simulink model "OpenLoop"  (R2022b)
settings: Solver=ode1  StartTime=0.0  StopTime=10  FixedStep=0.002  RelTol=1e-3  EnableMultiTasking=on
values from neighbouring files (symbols this model uses):
  a = -1/tau    (= -50)    [data_modele.m]
  Ao = [a 0;1 0]    [data_modele.m]
  Aobis = [a 0 b;1 0 0;0 0 0]    [data_modele.m]
  b = context.isCodeGenTarget('rtw')    [DCMotor1Set.m]    (also in DCMotor2Set.m; Enc1Period.m; Enc1Read.m; data_modele.m = 2500)
  Bo = [b;0]    [data_modele.m]
  Bobis = [b;0;0]    [data_modele.m]
  Co = [0 1]    [data_modele.m]
  Cobis = [0 1 0]    [data_modele.m]
  k1 = K(1, 2)    [data_modele.m]
  k2 = K(1, 1)    [data_modele.m]
  Kb = 50    [data_modele.m]
  L = transpose(Lt)    [data_modele.m]
  Lbis = transpose(Lbist)    [data_modele.m]
undefined symbols (not defined in the file or in its folder): sigbuilder_block
libraries: simulink x2
settings Model: SimulationMode=external  ExtModeTrigDuration=2  VariantFading=off  Creator=Alex  LastModifiedBy=mtroislo
settings SolverCC: AlgebraicLoopSolver=TrustRegion
settings DataIOCC: SaveFormat=StructureWithTime  ReturnWorkspaceOutputs=off
settings OptimizationCC: PassReuseOutputArgsAs=Individual arguments  MaxStackSize=64  EfficientTunableParamExpr=on
settings DebuggingCC: ParameterTunabilityLossMsg=error  UnconnectedInputMsg=warning  UnconnectedOutputMsg=warning  UnconnectedLineMsg=warning  SFMachineParentedDataDiag=warning  ArithmeticOperatorsInVariantConditions=warning
settings HardwareCC: ProdBitPerInt=16  ProdBitPerPointer=16  ProdBitPerSizeT=16  ProdBitPerPtrDiffT=16  ProdLargestAtomicFloat=None  ProdWordSize=8  ProdHWDeviceType=Atmel->AVR
settings ModelReferenceCC: EnableRefExpFcnMdlSchedulingChecks=on
settings SFSimCC: SimUseLocalCustomCode=off  MATLABDynamicMemAlloc=off  CustomCodeUndefinedFunction=UseInterfaceOnly
settings RTWCC: Description=Embedded Coder  SystemTargetFile=ert.tlc  HardwareBoard=Arduino Mega 2560  TLCOptions=-aInlineSetEventsForThisBaseRateFcn=TLC_FALSE -aSuppressMultiTaskScheduler=TLC_FALSE -aRateBasedStepFcn=1  TemplateMakefile=ert_default_tmf  RTWUseLocalCustomCode=off  Toolchain=Arduino AVR  BuildConfiguration=Faster Runs  IncludeHyperlinkInReport=on  DLArmComputeVersion=19.05
settings CodeAppCC: ForceParamTrailComments=on  IgnoreCustomStorageClasses=off  OperatorAnnotations=on  SimulinkDataObjDesc=on  SFDataObjDesc=on  InsertBlockDesc=on
settings ERTTargetCC: SupportContinuousTime=on  SupportVariableSizeSignals=on

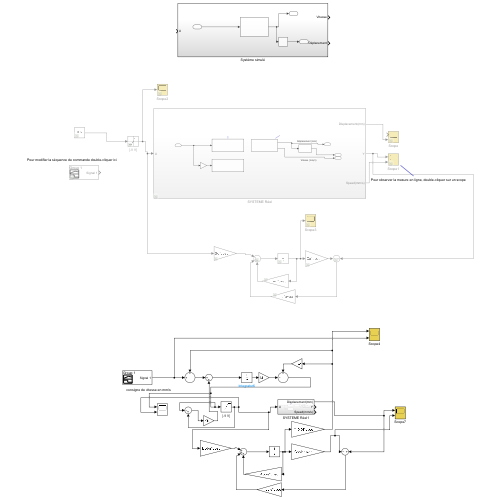
[thumbnail: Simulink's stored preview of the top-level diagram]
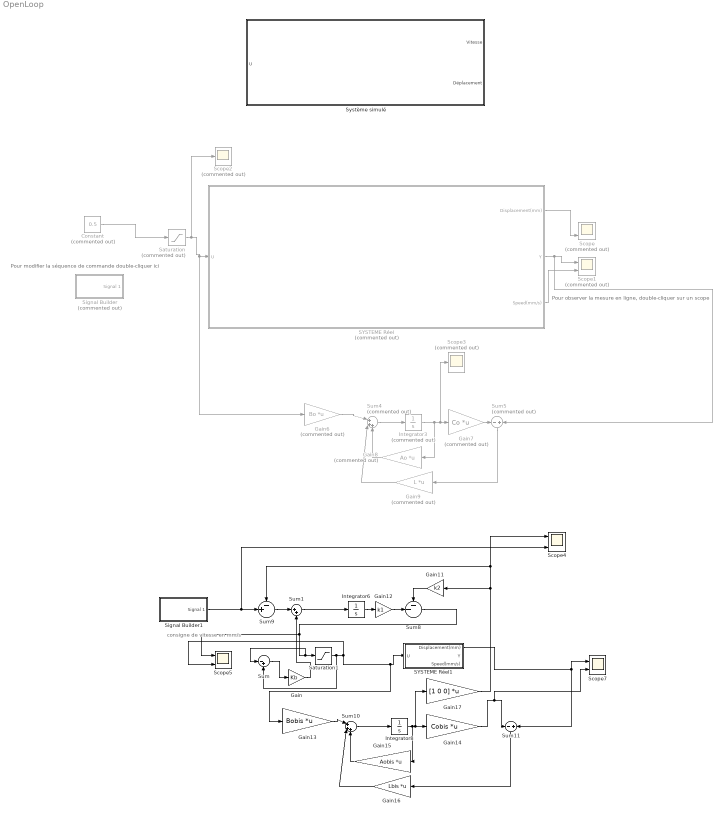
== system OpenLoop ==
  note: Pour observer la mesure en ligne, double-cliquer sur un scope
  note: Pour modifier la séquence de commande double-cliquer ici
  note: consigne de vitesse en mm/s
  Constant : Constant  Commented=on  Value=0.5
  Gain : Gain  Gain=Kb
  Gain11 : Gain  Gain=k2
  Gain12 : Gain  Gain=k1
  Gain13 : Gain  Gain=Bobis  Multiplication=Matrix(K*u) (u vector)
  Gain14 : Gain  Gain=Cobis  Multiplication=Matrix(K*u) (u vector)
  Gain15 : Gain  Gain=Aobis  Multiplication=Matrix(K*u) (u vector)
  Gain16 : Gain  Gain=Lbis  Multiplication=Matrix(K*u) (u vector)
  Gain17 : Gain  Gain=[1 0 0]  Multiplication=Matrix(K*u) (u vector)
  Gain6 : Gain  Commented=on  Gain=Bo  Multiplication=Matrix(K*u) (u vector)
  Gain7 : Gain  Commented=on  Gain=Co  Multiplication=Matrix(K*u) (u vector)
  Gain8 : Gain  Commented=on  Gain=Ao  Multiplication=Matrix(K*u) (u vector)
  Gain9 : Gain  Commented=on  Gain=L  Multiplication=Matrix(K*u) (u vector)
  Integrator3 : Integrator  Commented=on
  Integrator6 : Integrator
  Integrator8 : Integrator
  SYSTEME Réel : Subsystem  Commented=on
  SYSTEME Réel1 : Subsystem
  Saturation : Saturate  Commented=on  UpperLimit=9  LowerLimit=-9
      settings: AttributesFormatString=[%<LowerLimit> %<UpperLimit>]
  Saturation1 : Saturate  UpperLimit=9  LowerLimit=-9
      settings: AttributesFormatString=[%<LowerLimit> %<UpperLimit>]
  Scope : Scope  Commented=on  NumInputPorts=2
  Scope1 : Scope  Commented=on  NumInputPorts=2
  Scope2 : Scope  Commented=on
  Scope3 : Scope  Commented=on
  Scope4 : Scope  NumInputPorts=2
  Scope5 : Scope  NumInputPorts=2
  Scope7 : Scope  NumInputPorts=2
  Signal Builder : Subsystem  Tag=STV Subsys  Commented=on  LoadFcn=sigbuilder_block('load');  StartFcn=sigbuilder_block('start');  StopFcn=sigbuilder_block('stop');  ClipboardFcn=sigbuilder_block('clipboard');  mask(Sigbuilder block){tuvar=[0:10]}
      mask help: Simulink:masks:SigbuilderBlock_MD
      mask init:
      | if ~strcmp(get_param(bdroot(gcbh),'SimulationStatus'),'stopped') tuvar = sigbuilder_block('maskInit'); end
      settings: CopyFcn=sigbuilder_block('copy');  DeleteFcn=sigbuilder_block('delete');  ModelCloseFcn=sigbuilder_block('modelClose');  PreSaveFcn=sigbuilder_block('preSave');  PauseFcn=sigbuilder_block('pause');  ContinueFcn=sigbuilder_block('continue');  NameChangeFcn=sigbuilder_block('namechange');  OpenFcn=sigbuilder_block('open',[382.125 217.125 550.5 400.5 ]);  CloseFcn=sigbuilder_block('close');
      mask Display: plot(0, 0, 100, 100,[2, 2, 32, 32, 2], [68, 8, 8, 68, 68],[32, 2], [38, 38], [32, 19, 2],[53, 60, 44], [32, 17, 17, 2],[16, 16, 31, 31]);txt = getActiveGroup(gcbh);text(2, 100, txt,'verticalAlignment', 'top');
  Signal Builder1 : Subsystem  Tag=STV Subsys  LoadFcn=sigbuilder_block('load',[437.6 199.2 550.4 400 ]);  StartFcn=sigbuilder_block('start');  StopFcn=sigbuilder_block('stop');  ClipboardFcn=sigbuilder_block('clipboard');  mask(Sigbuilder block){tuvar=[0:10]}
      mask help: Simulink:masks:SigbuilderBlock_MD
      mask init:
      | if ~strcmp(get_param(bdroot(gcbh),'SimulationStatus'),'stopped') tuvar = sigbuilder_block('maskInit'); end
      settings: CopyFcn=sigbuilder_block('copy');  DeleteFcn=sigbuilder_block('delete');  ModelCloseFcn=sigbuilder_block('modelClose');  PreSaveFcn=sigbuilder_block('preSave');  PauseFcn=sigbuilder_block('pause');  ContinueFcn=sigbuilder_block('continue');  NameChangeFcn=sigbuilder_block('namechange');  OpenFcn=sigbuilder_block('open',[437.6 199.2 550.4 400 ]);  CloseFcn=sigbuilder_block('close');
      mask Display: plot(0, 0, 100, 100,[2, 2, 32, 32, 2], [68, 8, 8, 68, 68],[32, 2], [38, 38], [32, 19, 2],[53, 60, 44], [32, 17, 17, 2],[16, 16, 31, 31]);txt = getActiveGroup(gcbh);text(2, 100, txt,'verticalAlignment', 'top');
  Sum : Sum  Inputs=|-+
  Sum1 : Sum  Inputs=|++
  Sum10 : Sum  Inputs=|+++
  Sum11 : Sum  Inputs=-|+
  Sum4 : Sum  Commented=on  Inputs=|+++
  Sum5 : Sum  Commented=on  Inputs=-|+
  Sum8 : Sum  Inputs=--|
  Sum9 : Sum  Inputs=-+|
  Système simulé : Subsystem
  wires:
  SYSTEME Réel/1(Displacement(mm)) -> Scope/2
  SYSTEME Réel/2(Y) -> Sum5/2, Scope1/1
  SYSTEME Réel/3(Speed(mm/s)) -> Scope1/2
  Gain7/1 -> Sum5/1
  Gain9/1 -> Sum4/2
  Gain8/1 -> Sum4/3
  Sum5/1 -> Gain9/1
  Sum4/1 -> Integrator3/1
  Gain6/1 -> Sum4/1
  Integrator3/1 -> Gain8/1, Scope3/1, Gain7/1
  Saturation/1 -> SYSTEME Réel/1(U), Gain6/1, Scope2/1
  Constant/1 -> Saturation/1
  Sum11/1 -> Gain16/1
  Gain13/1 -> Sum10/1
  Gain16/1 -> Sum10/2
  Gain14/1 -> Scope7/2, Sum11/1
  Sum10/1 -> Integrator8/1
  Gain11/1 -> Sum8/1
  Gain15/1 -> Sum10/3
  Gain12/1 -> Sum8/2
  Gain17/1 -> Scope4/1, Sum9/1, Gain11/1
  SYSTEME Réel1/1(Displacement(mm)) -> Scope7/1, Sum11/2
  Integrator8/1 -> Gain15/1, Gain17/1, Gain14/1
  Integrator6/1 -> Gain12/1
  Signal Builder1/1(Signal 1) -> Scope4/2, Sum9/2
  Sum8/1 -> Scope5/1, Sum/1, Saturation1/1
  Saturation1/1 -> Sum/2, Gain13/1, SYSTEME Réel1/1(U), Scope5/2
  Sum/1 -> Gain/1
  Sum9/1 -> Sum1/1
  Sum1/1 -> Integrator6/1
  Gain/1 -> Sum1/2

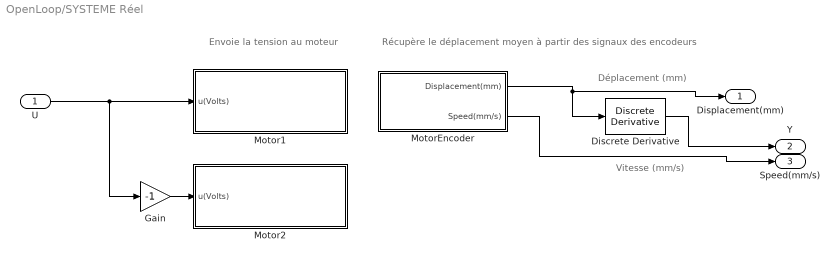
== system OpenLoop/SYSTEME Réel ==
  note: Déplacement (mm)
  note: Vitesse (mm/s)
  note: Récupère le déplacement moyen à partir des signaux des encodeurs
  note: Envoie la tension au moteur
  U : Inport
  Discrete Derivative : simulink/Discrete/Discrete Derivative  gainval=1.0  ICPrevScaledInput=0.0  OutMin=[]  OutMax=[]  OutDataType=fixdt(1, 16)  OutScaling=2^-10  DoSatur=off
  Gain : Gain  Gain=-1
  Motor1 : Subsystem  mask{Vmax=12}
      mask prompts: Vmax "Power supply Voltage"
  Motor2 : Subsystem  mask{Vmax=12}
      mask prompts: Vmax "Power supply Voltage"
  MotorEncoder : Subsystem  mask{pulsePerTurn=8, beltPitch=2.032, nTeeth=90, gearRatio=46}
      mask prompts: pulsePerTurn "Encoder resolution"; beltPitch "Belt Pitch"; nTeeth "Number of teeth"; gearRatio "Gear ratio"
  Displacement(mm) : Outport
  Y : Outport  Port=2
  Speed(mm/s) : Outport  Port=3
  wires:
  U/1 -> Gain/1, Motor1/1(u(Volts))
  Discrete Derivative/1 -> Y/1
  Gain/1 -> Motor2/1(u(Volts))
  MotorEncoder/1(Displacement(mm)) -> Displacement(mm)/1, Discrete Derivative/1
  MotorEncoder/2(Speed(mm/s)) -> Speed(mm/s)/1

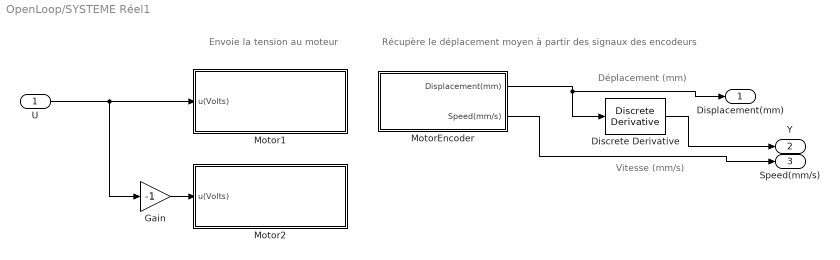
== system OpenLoop/SYSTEME Réel1 ==
  note: Déplacement (mm)
  note: Vitesse (mm/s)
  note: Récupère le déplacement moyen à partir des signaux des encodeurs
  note: Envoie la tension au moteur
  U : Inport
  Discrete Derivative : simulink/Discrete/Discrete Derivative  gainval=1.0  ICPrevScaledInput=0.0  OutMin=[]  OutMax=[]  OutDataType=fixdt(1, 16)  OutScaling=2^-10  DoSatur=off
  Gain : Gain  Gain=-1
  Motor1 : Subsystem  mask{Vmax=12}
      mask prompts: Vmax "Power supply Voltage"
  Motor2 : Subsystem  mask{Vmax=12}
      mask prompts: Vmax "Power supply Voltage"
  MotorEncoder : Subsystem  mask{pulsePerTurn=8, beltPitch=2.032, nTeeth=90, gearRatio=46}
      mask prompts: pulsePerTurn "Encoder resolution"; beltPitch "Belt Pitch"; nTeeth "Number of teeth"; gearRatio "Gear ratio"
  Displacement(mm) : Outport
  Y : Outport  Port=2
  Speed(mm/s) : Outport  Port=3
  wires:
  U/1 -> Gain/1, Motor1/1(u(Volts))
  Discrete Derivative/1 -> Y/1
  Gain/1 -> Motor2/1(u(Volts))
  MotorEncoder/1(Displacement(mm)) -> Displacement(mm)/1, Discrete Derivative/1
  MotorEncoder/2(Speed(mm/s)) -> Speed(mm/s)/1

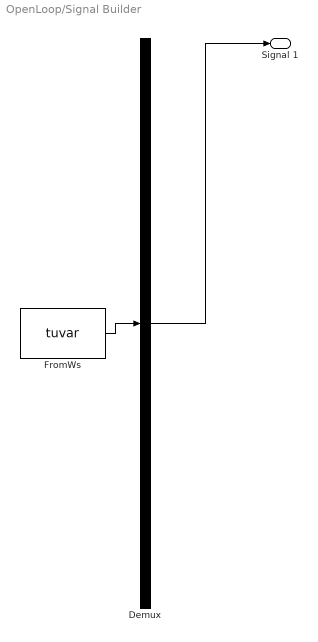
== system OpenLoop/Signal Builder ==
  Demux : Demux  Tag=STV Demux  Outputs=1
      settings: DisplayOption=none
  FromWs : FromWorkspace  Tag=STV FromWs  VariableName=tuvar
      SigBuilderData=|
      | common.afterFinalStr = 'Extrapolate'
      | common.sampleTime = 0
      | dataSet.timeRange = [0 10]
      | dataSet.name = 'Group 1'
      | sbobj.Groups.Name = 'Group 1'
      | sbobj.Groups.Signals.Name = 'Signal 1'
      | sbobj.Groups.Signals.XData = [0 1 1 1.5 1.5 4 4 5 5 7 7 8 8 9 9 9.5 9.5 10]
      | sbobj.Groups.Signals.YData = [0 0 7 7 0 0 4 4 0 0 -4 -4 0 0 -7 -7 0 0]
  Signal 1 : Outport  Tag=STV Outport  VectorParamsAs1DForOutWhenUnconnected=off
  wires:
  Demux/1 -> Signal 1/1
  FromWs/1 -> Demux/1

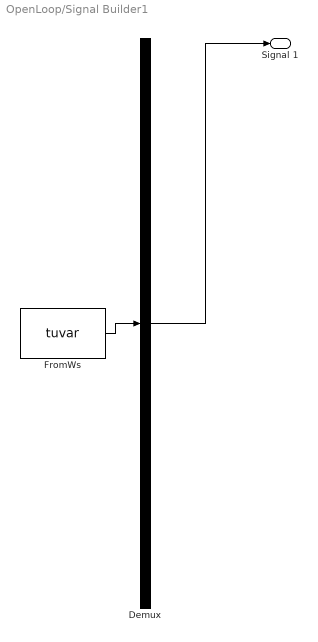
== system OpenLoop/Signal Builder1 ==
  Demux : Demux  Tag=STV Demux  Outputs=1
      settings: DisplayOption=none
  FromWs : FromWorkspace  Tag=STV FromWs  VariableName=tuvar
      SigBuilderData=|
      | common.afterFinalStr = 'Extrapolate'
      | common.sampleTime = 0
      | dataSet.timeRange = [0 10]
      | dataSet.name = 'Group 1'
      | sbobj.Groups.Name = 'Group 1'
      | sbobj.Groups.Signals.Name = 'Signal 1'
      | sbobj.Groups.Signals.XData = [0 4 4 5 5 10]
      | sbobj.Groups.Signals.YData = [250 250 700 700 250 250]
  Signal 1 : Outport  Tag=STV Outport
  wires:
  Demux/1 -> Signal 1/1
  FromWs/1 -> Demux/1

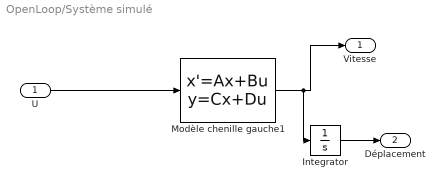
== system OpenLoop/Système simulé ==
  U : Inport
  Integrator : Integrator
  Modèle chenille gauche1 : StateSpace  A=a  B=b  D=0  InitialCondition=0
  Vitesse : Outport
  Déplacement : Outport  Port=2
  wires:
  U/1 -> Modèle chenille gauche1/1
  Modèle chenille gauche1/1 -> Integrator/1, Vitesse/1
  Integrator/1 -> Déplacement/1

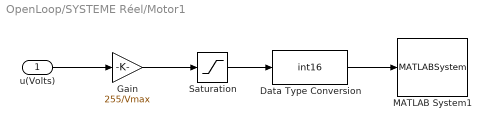
== system OpenLoop/SYSTEME Réel/Motor1 ==
  u(Volts) : Inport
  Data Type Conversion : DataTypeConversion  OutDataTypeStr=int16  SaturateOnIntegerOverflow=off  RndMeth=Floor
  Gain : Gain  Gain=255/Vmax
      settings: AttributesFormatString=%<Gain>
  MATLAB System1 : MATLABSystem  System=DCMotor1Set
      mask Type: DCMotor1Set
      mask Display:
      | disp('DC Motor 1');
      | port_label('input',1,'u');
  Saturation : Saturate  UpperLimit=255  LowerLimit=-255
  wires:
  Gain/1 -> Saturation/1
  u(Volts)/1 -> Gain/1
  Data Type Conversion/1 -> MATLAB System1/1
  Saturation/1 -> Data Type Conversion/1

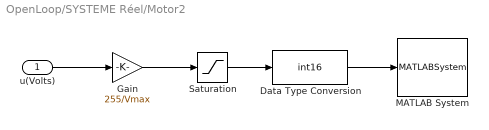
== system OpenLoop/SYSTEME Réel/Motor2 ==
  u(Volts) : Inport
  Data Type Conversion : DataTypeConversion  OutDataTypeStr=int16  SaturateOnIntegerOverflow=off  RndMeth=Floor
  Gain : Gain  Gain=255/Vmax
      settings: AttributesFormatString=%<Gain>
  MATLAB System : MATLABSystem  System=DCMotor2Set
      mask Type: DCMotor2Set
      mask Display:
      | disp('DC Motor 2');
      | port_label('input',1,'u');
  Saturation : Saturate  UpperLimit=255  LowerLimit=-255
  wires:
  Saturation/1 -> Data Type Conversion/1
  Data Type Conversion/1 -> MATLAB System/1
  u(Volts)/1 -> Gain/1
  Gain/1 -> Saturation/1

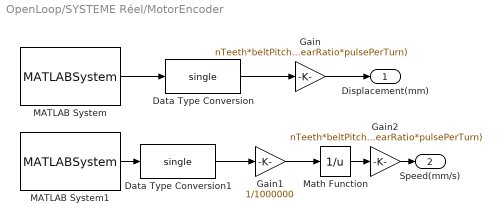
== system OpenLoop/SYSTEME Réel/MotorEncoder ==
  Data Type Conversion : DataTypeConversion  OutDataTypeStr=single  SaturateOnIntegerOverflow=off  RndMeth=Floor
  Data Type Conversion1 : DataTypeConversion  OutDataTypeStr=single  SaturateOnIntegerOverflow=off  RndMeth=Floor
  Gain : Gain  Gain=nTeeth*beltPitch/(gearRatio*pulsePerTurn)  OutDataTypeStr=single
      settings: AttributesFormatString=%<Gain>
  Gain1 : Gain  Gain=1/1000000
  Gain2 : Gain  Gain=nTeeth*beltPitch/(gearRatio*pulsePerTurn)  OutDataTypeStr=single
      settings: AttributesFormatString=%<Gain>
  MATLAB System : MATLABSystem  System=Enc1Read  SampleTime=0.002
      mask Type: Enc1Read
      mask Display:
      | disp('Encoder 1');
      | port_label('output',1,'y');
  MATLAB System1 : MATLABSystem  System=Enc1Period  SampleTime=0.002
      mask Type: Enc1Period
      mask Display:
      | disp('Encoder Period 1');
      | port_label('output',1,'y');
  Math Function : Math  Operator=reciprocal  SignedPower=on  OutputSignalType=real  OutDataTypeStr=single  SaturateOnIntegerOverflow=off
  Displacement(mm) : Outport  VectorParamsAs1DForOutWhenUnconnected=off
  Speed(mm/s) : Outport  Port=2  VectorParamsAs1DForOutWhenUnconnected=off
  wires:
  MATLAB System/1 -> Data Type Conversion/1
  Gain/1 -> Displacement(mm)/1
  Data Type Conversion/1 -> Gain/1
  Gain1/1 -> Math Function/1
  Data Type Conversion1/1 -> Gain1/1
  MATLAB System1/1 -> Data Type Conversion1/1
  Math Function/1 -> Gain2/1
  Gain2/1 -> Speed(mm/s)/1

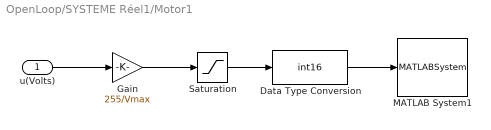
== system OpenLoop/SYSTEME Réel1/Motor1 ==
  u(Volts) : Inport
  Data Type Conversion : DataTypeConversion  OutDataTypeStr=int16  SaturateOnIntegerOverflow=off  RndMeth=Floor
  Gain : Gain  Gain=255/Vmax
      settings: AttributesFormatString=%<Gain>
  MATLAB System1 : MATLABSystem  System=DCMotor1Set
      mask Type: DCMotor1Set
      mask Display:
      | disp('DC Motor 1');
      | port_label('input',1,'u');
  Saturation : Saturate  UpperLimit=255  LowerLimit=-255
  wires:
  Gain/1 -> Saturation/1
  u(Volts)/1 -> Gain/1
  Data Type Conversion/1 -> MATLAB System1/1
  Saturation/1 -> Data Type Conversion/1

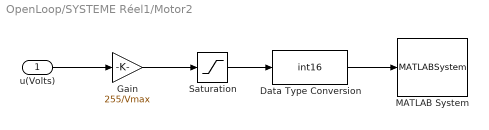
== system OpenLoop/SYSTEME Réel1/Motor2 ==
  u(Volts) : Inport
  Data Type Conversion : DataTypeConversion  OutDataTypeStr=int16  SaturateOnIntegerOverflow=off  RndMeth=Floor
  Gain : Gain  Gain=255/Vmax
      settings: AttributesFormatString=%<Gain>
  MATLAB System : MATLABSystem  System=DCMotor2Set
      mask Type: DCMotor2Set
      mask Display:
      | disp('DC Motor 2');
      | port_label('input',1,'u');
  Saturation : Saturate  UpperLimit=255  LowerLimit=-255
  wires:
  Saturation/1 -> Data Type Conversion/1
  Data Type Conversion/1 -> MATLAB System/1
  u(Volts)/1 -> Gain/1
  Gain/1 -> Saturation/1

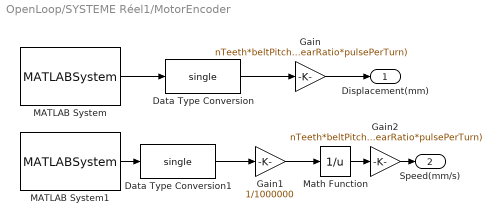
== system OpenLoop/SYSTEME Réel1/MotorEncoder ==
  Data Type Conversion : DataTypeConversion  OutDataTypeStr=single  SaturateOnIntegerOverflow=off  RndMeth=Floor
  Data Type Conversion1 : DataTypeConversion  OutDataTypeStr=single  SaturateOnIntegerOverflow=off  RndMeth=Floor
  Gain : Gain  Gain=nTeeth*beltPitch/(gearRatio*pulsePerTurn)  OutDataTypeStr=single
      settings: AttributesFormatString=%<Gain>
  Gain1 : Gain  Gain=1/1000000
  Gain2 : Gain  Gain=nTeeth*beltPitch/(gearRatio*pulsePerTurn)  OutDataTypeStr=single
      settings: AttributesFormatString=%<Gain>
  MATLAB System : MATLABSystem  System=Enc1Read  SampleTime=0.002
      mask Type: Enc1Read
      mask Display:
      | disp('Encoder 1');
      | port_label('output',1,'y');
  MATLAB System1 : MATLABSystem  System=Enc1Period  SampleTime=0.002
      mask Type: Enc1Period
      mask Display:
      | disp('Encoder Period 1');
      | port_label('output',1,'y');
  Math Function : Math  Operator=reciprocal  SignedPower=on  OutputSignalType=real  OutDataTypeStr=single  SaturateOnIntegerOverflow=off
  Displacement(mm) : Outport  VectorParamsAs1DForOutWhenUnconnected=off
  Speed(mm/s) : Outport  Port=2  VectorParamsAs1DForOutWhenUnconnected=off
  wires:
  MATLAB System/1 -> Data Type Conversion/1
  Gain/1 -> Displacement(mm)/1
  Data Type Conversion/1 -> Gain/1
  Gain1/1 -> Math Function/1
  Data Type Conversion1/1 -> Gain1/1
  MATLAB System1/1 -> Data Type Conversion1/1
  Math Function/1 -> Gain2/1
  Gain2/1 -> Speed(mm/s)/1
